simulink model "example_Hydraulic_FlowDiverter"  (R2013b)
settings: Solver=ode45  StartTime=0.0  StopTime=210  RelTol=1e-3
libraries: carnot x6, simulink x1
settings Model: Creator=drhf  LastModifiedBy=drhf
settings OptimizationCC: ExpressionDepthLimit=2147483647
settings DebuggingCC: StateNameClashWarn=warning
settings GRTTargetCC: CombineOutputUpdateFcns=off  GRTInterface=on

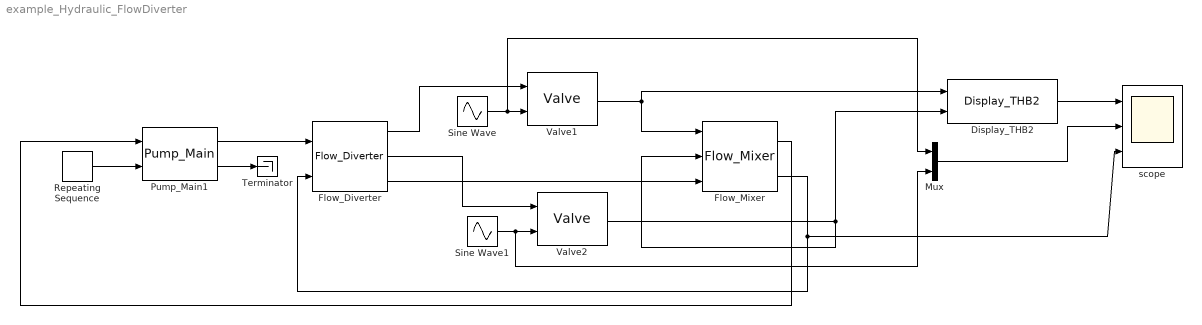
== system example_Hydraulic_FlowDiverter ==
  Display_THB2 : carnot/Outputs/Display_THB2  t=off  m=on  p=off  id=off  mix=off  d=off
  Flow_Diverter : carnot/Hydraulics/Flow_Diverter
  Flow_Mixer : carnot/Hydraulics/Flow_Mixer  t=1
  Mux : Mux  Inputs=2
  Pump_Main1 : carnot/Hydraulics/Pump_Main  a0=2.7e4  a1=-1.2e4  a2=0%-3e-3  dia=0.025  t1=5  p0=3e5  IDchk=off  fluid_id=Water  mix=0  ua=1  mcp=500  tamb=20
  Repeating Sequence : simulink/Sources/Repeating Sequence  rep_seq_t=[0 20 60 200]  rep_seq_y=[0 0 1 1]
  Sine Wave : Sin  Amplitude=0.6  Bias=0.5  Frequency=1/20  SampleTime=0
  Sine Wave1 : Sin  Amplitude=0.6  Bias=0.5  Frequency=1/20  Phase=pi  SampleTime=0
  Terminator : Terminator
  Valve1 : carnot/Hydraulics/Valve  pos_values=[0 0.1 1]  dp_values=[1e6 1e6 1]
  Valve2 : carnot/Hydraulics/Valve  pos_values=[0 0.1 1]  dp_values=[1e6 1e6 1]
  scope : Scope  NumInputPorts=3
      settings: TickLabels=on  YMin=0~-5~-5  YMax=5~5~5
  wires:
  Repeating Sequence/1 -> Pump_Main1/2
  Pump_Main1/2 -> Terminator/1
  Sine Wave/1 -> Mux/1, Valve1/2
  Pump_Main1/1 -> Flow_Diverter/1
  Flow_Diverter/1 -> Valve1/1
  Sine Wave1/1 -> Mux/2, Valve2/2
  Flow_Diverter/2 -> Valve2/1
  Flow_Diverter/3 -> Flow_Mixer/3
  Flow_Mixer/2 -> scope/3, Flow_Diverter/2
  Flow_Mixer/1 -> Pump_Main1/1
  Display_THB2/1 -> scope/1
  Mux/1 -> scope/2
  Valve1/1 -> Display_THB2/1, Flow_Mixer/1
  Valve2/1 -> Display_THB2/2, Flow_Mixer/2
